simulink model "PID_Controller"  (R2020a)
settings: Solver=VariableStepAuto  StartTime=0.0  StopTime=0.2  RelTol=1e-3
PostLoadFcn:
  | J = 3.2284E-6;
  | b = 3.5077E-6;
  | Ke = 0.0274;
  | Kt = 0.0274;
  | R = 4;
  | L = 2.75E-6;
settings Model: DataDictionary=w2p4vars.sldd  Creator=Anjali123  LastModifiedBy=Anjali123
settings DataIOCC: SaveOutput=off  SaveTime=off

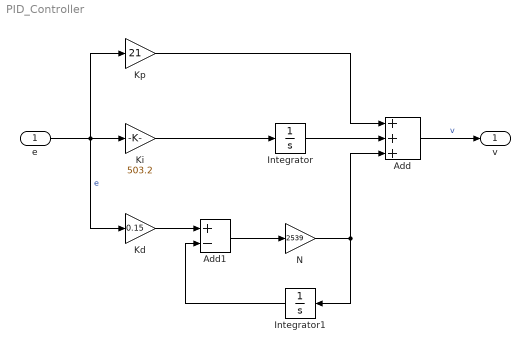
== system PID_Controller ==
  e : Inport  OutDataTypeStr=double  PortDimensions=1  SampleTime=0
  Add : Sum  Inputs=+++
  Add1 : Sum  Inputs=+-
  Integrator : Integrator
  Integrator1 : Integrator
  Kd : Gain  Gain=0.15
  Ki : Gain  Gain=503.2
  Kp : Gain  Gain=21
  N : Gain  Gain=2539
  v : Outport  OutDataTypeStr=double  PortDimensions=1  SampleTime=0
  wires:
  e/1 -> Kp/1, Ki/1, Kd/1  "e"
  Ki/1 -> Integrator/1
  Integrator/1 -> Add/2
  N/1 -> Add/3, Integrator1/1
  Kd/1 -> Add1/1
  Kp/1 -> Add/1
  Add/1 -> v/1  "v"
  Add1/1 -> N/1
  Integrator1/1 -> Add1/2
